simulink model "PROJECT_SIMULINK"  (R2024b)
settings: Solver=ode4  StartTime=t0  StopTime=tf  FixedStep=0.1  RelTol=1e-3
values from neighbouring files (symbols this model uses):
  a = 42000000    [PROJECT_SCRIPT.m]    (also in qmethod.m = 6844)
  ABN0 = diag([1, 1, 1])    [PROJECT_SCRIPT.m]    (also in qmethod.m)
  e = 0.1    [PROJECT_SCRIPT.m]    (also in qmethod.m = 0.0005568)
  G = 6.6743E-11    (= 6.6743e-11)    [PROJECT_SCRIPT.m]    (also in qmethod.m)
  H0 = sqrt(g01^2 + g11^2 + h11^2)    [PROJECT_SCRIPT.m]    (also in qmethod.m)
  i = 0.5    [PROJECT_SCRIPT.m]    (also in qmethod.m = deg2rad(97.36))
  J = diag([Ix, Iy, Iz])    [PROJECT_SCRIPT.m]    (also in qmethod.m = diag([0.0823, 0.0633, 0.0317]))
  jB = [0.01; 0.05; 0.01]    [PROJECT_SCRIPT.m]    (also in qmethod.m)
  Mt = 5.972E24    (= 5.972e+24)    [PROJECT_SCRIPT.m]    (also in qmethod.m)
  n = sqrt(G*Mt/a^3)    [PROJECT_SCRIPT.m]    (also in qmethod.m = 0.0011151076043)
  phi = deg2rad(11.5)    [PROJECT_SCRIPT.m]    (also in qmethod.m)
  RE = 6378000    [PROJECT_SCRIPT.m]    (also in qmethod.m = 6371000)
  theta0 = 0    [PROJECT_SCRIPT.m]    (also in qmethod.m)
  w0 = [wx0; wy0; wz0]    [PROJECT_SCRIPT.m]    (also in qmethod.m)
  wE = n    [PROJECT_SCRIPT.m]    (also in qmethod.m = 7.2921159e-05)
libraries: matrix_library x5
settings Model: Creator=esteb  LastModifiedBy=esteb

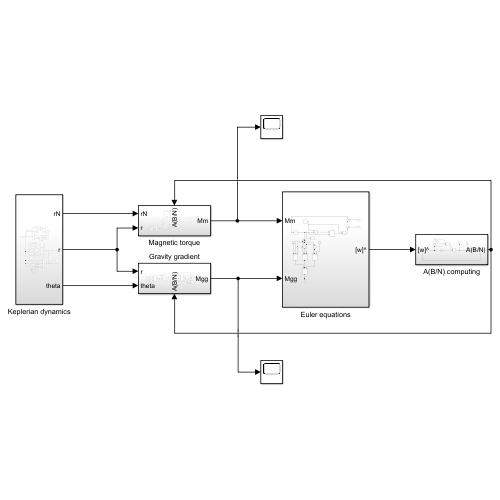
[thumbnail: Simulink's stored preview of the top-level diagram]
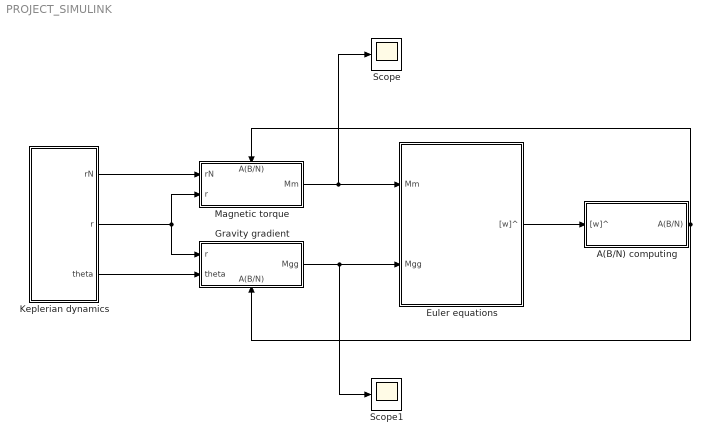
== system PROJECT_SIMULINK ==
  A(B/N) computing : Subsystem
  Euler equations : Subsystem
  Gravity gradient : Subsystem
      settings: PortSchema="{\"entries\":[{\"content\":{\"sides\":[{\"content\":{\"connectorIds\":[\"In1\",\"In2\"]},\"type\":\"ConnectorPlacement.EquallySpacedRectSide\",\"uuid\":\"c2d21b10-9a11-4d97-b795-06fc37f64ca8\"},{\"content\":{\"connectorIds\":[\"Out1\"],\"side\":\"RIGHT\"},\"type\":\"ConnectorPlacement.EquallySpacedRectSide\",\"uuid\":\"2995f645-6845-4ef4-adc0-5aa769d35de6\"},{\"content\":{\"side\":\"TOP\"},\"type\":\"ConnectorPlacement.EquallySpacedRectSide\",\"uuid\":\"22822c6c-8bba-432f-9ec4-c9bd815dca43\"},{\"content\":{\"connectorIds\":[\"In3\"],\"side\":\"BOTTOM\"},\"type\":\"ConnectorPlacement.EquallySpacedRectSide\",\"uuid\":\"1226eb0d-43f0-421d-ae78-502361aeaf7e\"}]},\"type\":\"ConnectorPlacement.EquallySpacedConnector\",\"uuid\":\"9a87865f-034e-4147-a08e-8e321d91c85d\"}],\"packageUris\":[\"http://schema.mathworks.com/mf0/Connector/R2020b\"],\"version\":\"1.0\"}"
  Keplerian dynamics : Subsystem
  Magnetic torque : Subsystem
      settings: PortSchema="{\"entries\":[{\"content\":{\"sides\":[{\"content\":{\"connectorIds\":[\"In1\",\"In2\"]},\"type\":\"ConnectorPlacement.EquallySpacedRectSide\",\"uuid\":\"c2d21b10-9a11-4d97-b795-06fc37f64ca8\"},{\"content\":{\"connectorIds\":[\"Out1\"],\"side\":\"RIGHT\"},\"type\":\"ConnectorPlacement.EquallySpacedRectSide\",\"uuid\":\"2995f645-6845-4ef4-adc0-5aa769d35de6\"},{\"content\":{\"connectorIds\":[\"In3\"],\"side\":\"TOP\"},\"type\":\"ConnectorPlacement.EquallySpacedRectSide\",\"uuid\":\"22822c6c-8bba-432f-9ec4-c9bd815dca43\"}]},\"type\":\"ConnectorPlacement.EquallySpacedConnector\",\"uuid\":\"9a87865f-034e-4147-a08e-8e321d91c85d\"}],\"packageUris\":[\"http://schema.mathworks.com/mf0/Connector/R2020b\"],\"version\":\"1.0\"}"
  Scope : Scope
  Scope1 : Scope
  wires:
  Magnetic torque/1(Mm) -> Euler equations/1(Mm), Scope/1
  Gravity gradient/1(Mgg) -> Euler equations/2(Mgg), Scope1/1
  Euler equations/1("[w]^") -> A(B/N) computing/1("[w]^")
  A(B/N) computing/1(A(B/N)) -> Gravity gradient/3(A(B/N)), Magnetic torque/3(A(B/N))
  Keplerian dynamics/1(rN) -> Magnetic torque/1(rN)
  Keplerian dynamics/3(theta) -> Gravity gradient/2(theta)
  Keplerian dynamics/2(r) -> Gravity gradient/1(r), Magnetic torque/2(r)

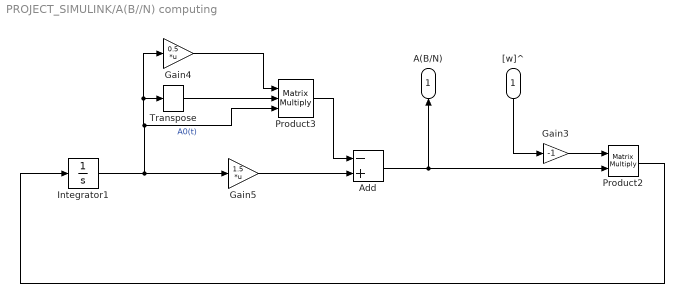
== system PROJECT_SIMULINK/A(B//N) computing ==
  "[w]^" : Inport
  Add : Sum  Inputs=-+
  Gain3 : Gain  Gain=-1
  Gain4 : Gain  Gain=0.5  Multiplication=Matrix(K*u)
  Gain5 : Gain  Gain=1.5  Multiplication=Matrix(K*u)
  Integrator1 : Integrator  InitialCondition=ABN0
  Product2 : Product  Multiplication=Matrix(*)
  Product3 : Product  Inputs=3  Multiplication=Matrix(*)
  Transpose : matrix_library/Transpose
  A(B/N) : Outport
  wires:
  Gain3/1 -> Product2/1
  Product3/1 -> Add/1
  Gain4/1 -> Product3/1
  Product2/1 -> Integrator1/1
  "[w]^"/1 -> Gain3/1
  Gain5/1 -> Add/2
  Add/1 -> A(B/N)/1, Product2/2
  Transpose/1 -> Product3/2
  Integrator1/1 -> Product3/3, Transpose/1, Gain4/1, Gain5/1  "A0(t)"

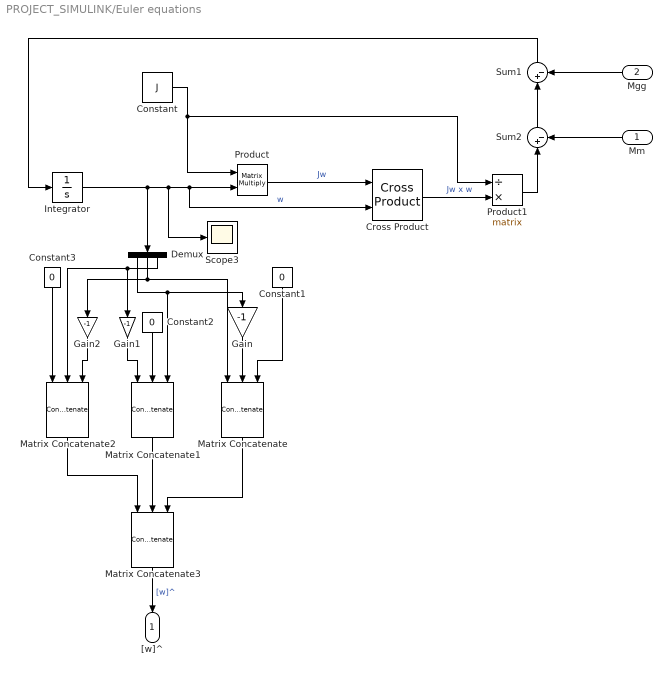
== system PROJECT_SIMULINK/Euler equations ==
  Mm : Inport
  Mgg : Inport  Port=2
  Constant : Constant  Value=J
  Constant1 : Constant  Value=0
  Constant2 : Constant  Value=0
  Constant3 : Constant  Value=0
  Cross Product : matrix_library/Cross Product
  Demux : Demux  Outputs=3
  Gain : Gain  Gain=-1
  Gain1 : Gain  Gain=-1
  Gain2 : Gain  Gain=-1
  Integrator : Integrator  InitialCondition=w0
  Matrix Concatenate : Concatenate  NumInputs=3  Mode=Multidimensional array
  Matrix Concatenate1 : Concatenate  NumInputs=3  Mode=Multidimensional array
  Matrix Concatenate2 : Concatenate  NumInputs=3  Mode=Multidimensional array
  Matrix Concatenate3 : Concatenate  NumInputs=3  Mode=Multidimensional array  ConcatenateDimension=2
  Product : Product  Multiplication=Matrix(*)
  Product1 : Product  Inputs=/*  Multiplication=Matrix(*)
  Scope3 : Scope
  Sum1 : Sum  Inputs=|+-
  Sum2 : Sum  Inputs=|+-
  "[w]^" : Outport
  wires:
  Matrix Concatenate2/1 -> Matrix Concatenate3/1
  Mgg/1 -> Sum1/2
  Product/1 -> Cross Product/1  "Jw"
  Demux/3 -> Matrix Concatenate2/2, Gain1/1
  Sum1/1 -> Integrator/1
  Cross Product/1 -> Product1/2  "Jw x w"
  Sum2/1 -> Sum1/1
  Constant/1 -> Product1/1, Product/1
  Constant1/1 -> Matrix Concatenate/3
  Matrix Concatenate/1 -> Matrix Concatenate3/3
  Constant2/1 -> Matrix Concatenate1/2
  Gain2/1 -> Matrix Concatenate2/3
  Integrator/1 -> Demux/1, Scope3/1, Cross Product/2, Product/2  "w"
  Matrix Concatenate1/1 -> Matrix Concatenate3/2
  Matrix Concatenate3/1 -> "[w]^"/1  "[w]^"
  Product1/1 -> Sum2/1
  Gain/1 -> Matrix Concatenate/2
  Demux/1 -> Matrix Concatenate1/3, Gain/1
  Demux/2 -> Gain2/1, Matrix Concatenate/1
  Constant3/1 -> Matrix Concatenate2/1
  Gain1/1 -> Matrix Concatenate1/1
  Mm/1 -> Sum2/2

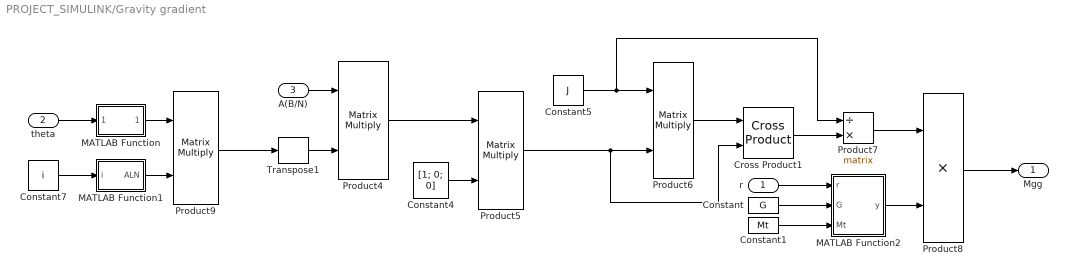
== system PROJECT_SIMULINK/Gravity gradient ==
  r : Inport
  theta : Inport  Port=2
  A(B/N) : Inport  Port=3
  Constant : Constant  Value=G
  Constant1 : Constant  Value=Mt
  Constant4 : Constant  Value=[1; 0; 0]
  Constant5 : Constant  Value=J
  Constant7 : Constant  Value=i
  Cross Product1 : matrix_library/Cross Product
  MATLAB Function : MATLAB Function  TreatAsAtomicUnit=on
  MATLAB Function1 : MATLAB Function  TreatAsAtomicUnit=on
  MATLAB Function2 : MATLAB Function  TreatAsAtomicUnit=on
  Product{4..6,9} (4 alike) : Product  Multiplication=Matrix(*)
  Product7 : Product  Inputs=/*  Multiplication=Matrix(*)
  Product8 : Product
  Transpose1 : matrix_library/Transpose
  Mgg : Outport
  wires:
  Product7/1 -> Product8/1
  Product9/1 -> Transpose1/1
  MATLAB Function1/1(ALN) -> Product9/2
  Product5/1 -> Cross Product1/2, Product6/2
  Cross Product1/1 -> Product7/2
  Constant7/1 -> MATLAB Function1/1(i)
  Constant5/1 -> Product7/1, Product6/1
  MATLAB Function2/1(y) -> Product8/2
  Transpose1/1 -> Product4/2
  Constant4/1 -> Product5/2
  Product4/1 -> Product5/1
  A(B/N)/1 -> Product4/1
  theta/1 -> MATLAB Function/1(theta)
  Product6/1 -> Cross Product1/1
  MATLAB Function/1(ALN) -> Product9/1
  r/1 -> MATLAB Function2/1(r)
  Product8/1 -> Mgg/1
  Constant1/1 -> MATLAB Function2/3(Mt)
  Constant/1 -> MATLAB Function2/2(G)

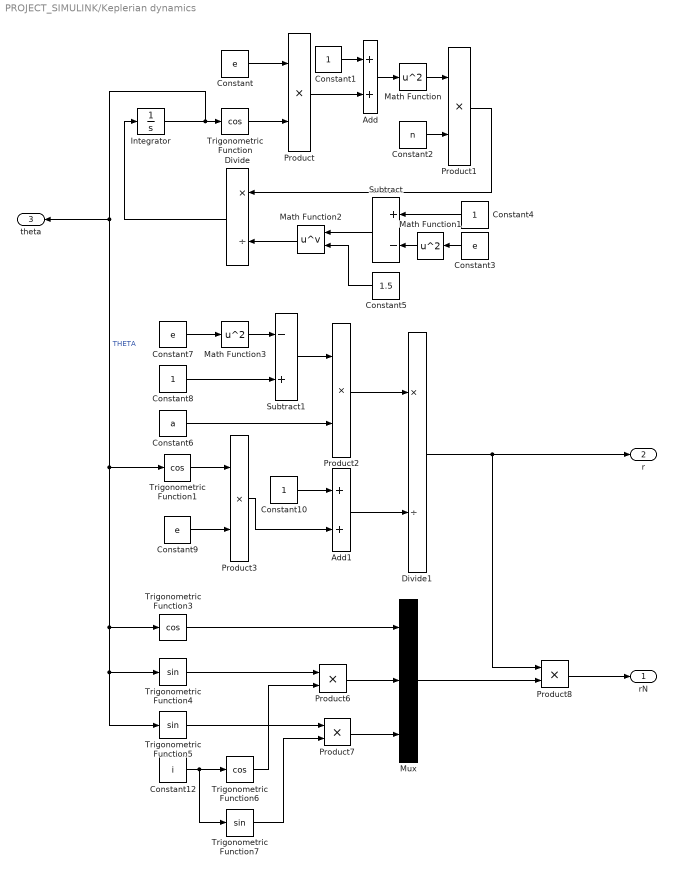
== system PROJECT_SIMULINK/Keplerian dynamics ==
  Add : Sum
  Add1 : Sum
  Constant{,3,7,9} (4 alike) : Constant  Value=e
  Constant{1,4,8,10} (4 alike) : Constant
  Constant12 : Constant  Value=i
  Constant2 : Constant  Value=n
  Constant5 : Constant  Value=1.5
  Constant6 : Constant  Value=a
  Divide : Product  Inputs=*/
  Divide1 : Product  Inputs=*/
  Integrator : Integrator  InitialCondition=theta0
  Math Function : Math  Operator=square
  Math Function1 : Math  Operator=square
  Math Function2 : Math  Operator=pow
  Math Function3 : Math  Operator=square
  Mux : Mux  Inputs=3
  Product{,1..3,6..8} (7 alike) : Product
  Subtract : Sum  Inputs=+-
  Subtract1 : Sum  Inputs=-+
  Trigonometric Function{,1,3,6} (4 alike) : Trigonometry  Operator=cos
  Trigonometric Function4 : Trigonometry
  Trigonometric Function5 : Trigonometry
  Trigonometric Function7 : Trigonometry
  rN : Outport
  r : Outport  Port=2
  theta : Outport  Port=3
  wires:
  Add/1 -> Math Function/1
  Trigonometric Function1/1 -> Product3/1
  Constant8/1 -> Subtract1/2
  Add1/1 -> Divide1/2
  Divide1/1 -> Product8/1, r/1
  Product3/1 -> Add1/2
  Product6/1 -> Mux/2
  Subtract/1 -> Math Function2/1
  Constant7/1 -> Math Function3/1
  Constant5/1 -> Math Function2/2
  Math Function2/1 -> Divide/2
  Product7/1 -> Mux/3
  Mux/1 -> Product8/2
  Product8/1 -> rN/1
  Constant4/1 -> Subtract/1
  Math Function1/1 -> Subtract/2
  Constant12/1 -> Trigonometric Function7/1, Trigonometric Function6/1
  Integrator/1 -> theta/1, Trigonometric Function5/1, Trigonometric Function4/1, Trigonometric Function3/1, Trigonometric Function1/1, Trigonometric Function/1  "THETA"
  Product1/1 -> Divide/1
  Trigonometric Function/1 -> Product/2
  Product2/1 -> Divide1/1
  Trigonometric Function5/1 -> Product7/1
  Subtract1/1 -> Product2/1
  Math Function/1 -> Product1/1
  Math Function3/1 -> Subtract1/1
  Trigonometric Function7/1 -> Product7/2
  Trigonometric Function6/1 -> Product6/2
  Constant1/1 -> Add/1
  Product/1 -> Add/2
  Constant9/1 -> Product3/2
  Trigonometric Function4/1 -> Product6/1
  Constant3/1 -> Math Function1/1
  Constant10/1 -> Add1/1
  Constant6/1 -> Product2/2
  Trigonometric Function3/1 -> Mux/1
  Constant2/1 -> Product1/2
  Divide/1 -> Integrator/1
  Constant/1 -> Product/1

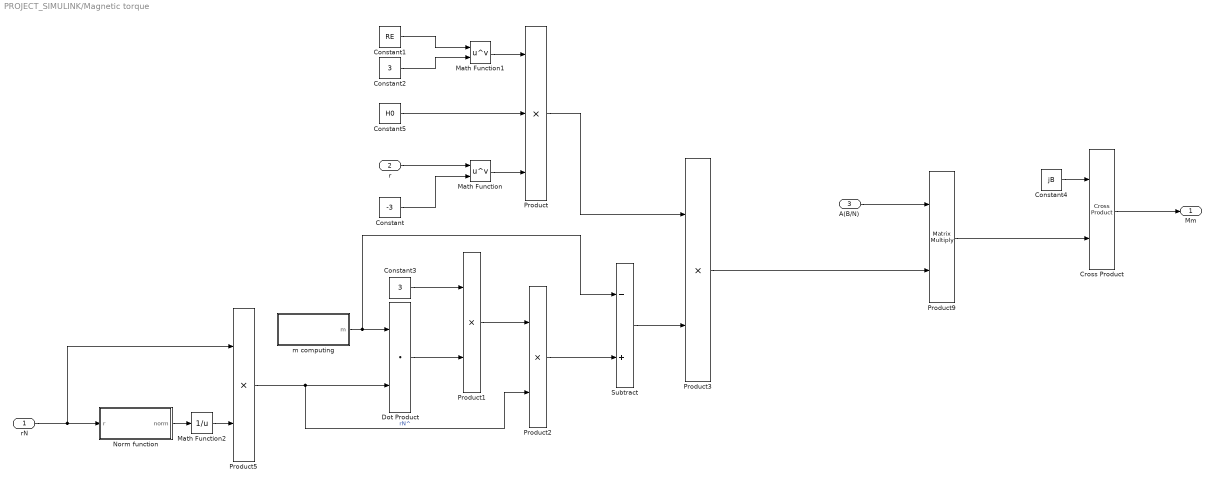
== system PROJECT_SIMULINK/Magnetic torque ==
  rN : Inport
  r : Inport  Port=2
  A(B/N) : Inport  Port=3
  Constant : Constant  Value=-3
  Constant1 : Constant  Value=RE
  Constant2 : Constant  Value=3
  Constant3 : Constant  Value=3
  Constant4 : Constant  Value=jB
  Constant5 : Constant  Value=H0
  Cross Product : matrix_library/Cross Product
  Dot Product : DotProduct  OutDataTypeStr=Inherit: Inherit via internal rule
  Math Function : Math  Operator=pow
  Math Function1 : Math  Operator=pow
  Math Function2 : Math  Operator=reciprocal
  Norm function : Subsystem
  Product : Product  Inputs=3
  Product{1..3,5} (4 alike) : Product
  Product9 : Product  Multiplication=Matrix(*)
  Subtract : Sum  Inputs=-+
  m computing : Subsystem
  Mm : Outport
  wires:
  Constant5/1 -> Product/2
  Constant3/1 -> Product1/1
  Product3/1 -> Product9/2
  Cross Product/1 -> Mm/1
  Math Function1/1 -> Product/1
  Product/1 -> Product3/1
  Product1/1 -> Product2/1
  Math Function2/1 -> Product5/2
  Constant/1 -> Math Function/2
  Dot Product/1 -> Product1/2
  Product5/1 -> Dot Product/2, Product2/2  "rN^"
  Constant1/1 -> Math Function1/1
  Product9/1 -> Cross Product/2
  Constant2/1 -> Math Function1/2
  Product2/1 -> Subtract/2
  rN/1 -> Product5/1, Norm function/1(r)
  Norm function/1(norm) -> Math Function2/1
  A(B/N)/1 -> Product9/1
  Constant4/1 -> Cross Product/1
  r/1 -> Math Function/1
  m computing/1(m) -> Dot Product/1, Subtract/1
  Math Function/1 -> Product/3
  Subtract/1 -> Product3/2

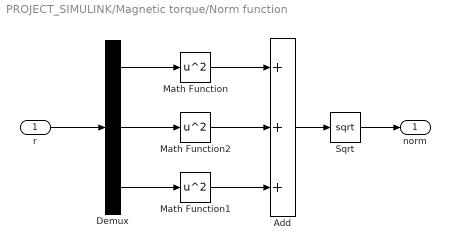
== system PROJECT_SIMULINK/Magnetic torque/Norm function ==
  r : Inport
  Add : Sum  Inputs=+++
  Demux : Demux  Outputs=3
  Math Function : Math  Operator=square
  Math Function1 : Math  Operator=square
  Math Function2 : Math  Operator=square
  Sqrt : Sqrt
  norm : Outport
  wires:
  r/1 -> Demux/1
  Math Function2/1 -> Add/2
  Math Function1/1 -> Add/3
  Math Function/1 -> Add/1
  Add/1 -> Sqrt/1
  Sqrt/1 -> norm/1
  Demux/1 -> Math Function/1
  Demux/2 -> Math Function2/1
  Demux/3 -> Math Function1/1

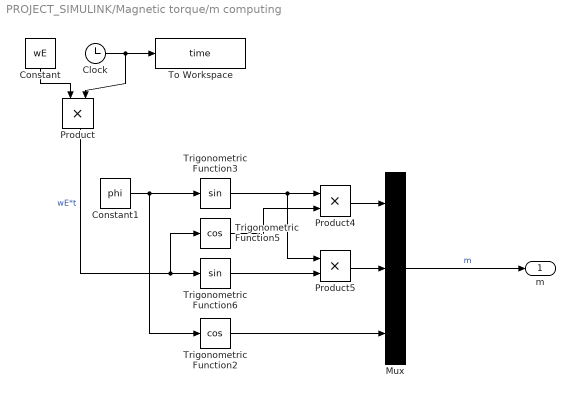
== system PROJECT_SIMULINK/Magnetic torque/m computing ==
  Clock : Clock
  Constant : Constant  Value=wE
  Constant1 : Constant  Value=phi
  Mux : Mux  Inputs=3
  Product : Product
  Product4 : Product
  Product5 : Product
  To Workspace : ToWorkspace  VariableName=time  SaveFormat=Timeseries  SampleTime=-1
  Trigonometric Function2 : Trigonometry  Operator=cos
  Trigonometric Function3 : Trigonometry
  Trigonometric Function5 : Trigonometry  Operator=cos
  Trigonometric Function6 : Trigonometry
  m : Outport
  wires:
  Constant1/1 -> Trigonometric Function2/1, Trigonometric Function3/1
  Clock/1 -> Product/2, To Workspace/1
  Mux/1 -> m/1  "m"
  Product/1 -> Trigonometric Function5/1, Trigonometric Function6/1  "wE*t"
  Trigonometric Function5/1 -> Product4/2
  Product4/1 -> Mux/1
  Trigonometric Function6/1 -> Product5/2
  Trigonometric Function3/1 -> Product5/1, Product4/1
  Product5/1 -> Mux/2
  Constant/1 -> Product/1
  Trigonometric Function2/1 -> Mux/3

== matlab function PROJECT_SIMULINK/Gravity gradient/MATLAB Function ==
  data: theta input; ALN output
function ALN = fcn(theta)
    ALN = [cos(theta), sin(theta), 0;
            -sin(theta), cos(theta), 0;
            0, 0, 1];
end

== matlab function PROJECT_SIMULINK/Gravity gradient/MATLAB Function1 ==
  data: i input; ALN output
function ALN = fcn(i)
    ALN = [1, 0, 0;
              0, cos(i), sin(i);
            0, -sin(i), cos(i)];
end

== matlab function PROJECT_SIMULINK/Gravity gradient/MATLAB Function2 ==
  data: r input; y output; G input; Mt input
function y = fcn(r,G,Mt)

y = 3*G*Mt/r^3;
